simulink library "csc_gnd_sta_lib"  (R2014b)
settings: Solver=ode45  StartTime=0.0  StopTime=10.0  RelTol=1e-3
undefined symbols (not defined in the file): scenario_data_dir
libraries: util_info_lib x1
settings Model: Creator=mstewart  LastModifiedBy=mstewart

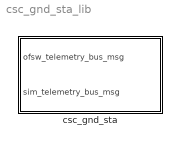
== system csc_gnd_sta_lib ==
  csc_gnd_sta : Subsystem  mask{dir_name=scenario_data_dir}
      mask prompts: dir_name "File Destination Directory (include '')"
      mask init:
      | csc_gnd_sta_callback(gcb, dir_name);
      mask Display:
      | color('blue');
      | text(0.02,0.05,'MoonEx', ...
      |  	'HorizontalAlignment','Left', ...
      | 	'VerticalAlignment','Bottom');

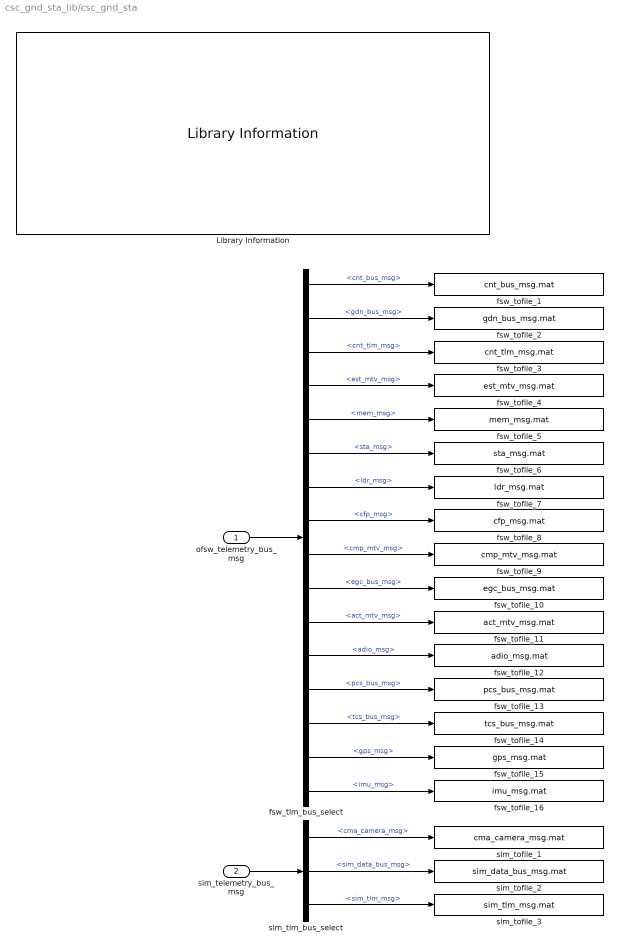
== system csc_gnd_sta_lib/csc_gnd_sta ==
  ofsw_telemetry_bus_msg : Inport
  sim_telemetry_bus_msg : Inport  Port=2
  Library Information : util_info_lib/Library Information  owner='NONE'
  fsw_tlm_bus_select : BusSelector  OutputSignals=cnt_bus_msg,gdn_bus_msg,cnt_tlm_msg,est_mtv_msg,mem_msg,sta_msg,ldr_msg,cfp_msg,cmp_mtv_msg,egc_bus_msg,act_mtv_msg,adio_msg,pcs_bus_msg,tcs_bus_msg,gps_msg,imu_msg
  fsw_tofile_1 : ToFile  Filename=cnt_bus_msg.mat  MatrixName=data  SaveFormat=Timeseries
  fsw_tofile_10 : ToFile  Filename=egc_bus_msg.mat  MatrixName=data  SaveFormat=Timeseries
  fsw_tofile_11 : ToFile  Filename=act_mtv_msg.mat  MatrixName=data  SaveFormat=Timeseries
  fsw_tofile_12 : ToFile  Filename=adio_msg.mat  MatrixName=data  SaveFormat=Timeseries
  fsw_tofile_13 : ToFile  Filename=pcs_bus_msg.mat  MatrixName=data  SaveFormat=Timeseries
  fsw_tofile_14 : ToFile  Filename=tcs_bus_msg.mat  MatrixName=data  SaveFormat=Timeseries
  fsw_tofile_15 : ToFile  Filename=gps_msg.mat  MatrixName=data  SaveFormat=Timeseries
  fsw_tofile_16 : ToFile  Filename=imu_msg.mat  MatrixName=data  SaveFormat=Timeseries
  fsw_tofile_2 : ToFile  Filename=gdn_bus_msg.mat  MatrixName=data  SaveFormat=Timeseries
  fsw_tofile_3 : ToFile  Filename=cnt_tlm_msg.mat  MatrixName=data  SaveFormat=Timeseries
  fsw_tofile_4 : ToFile  Filename=est_mtv_msg.mat  MatrixName=data  SaveFormat=Timeseries
  fsw_tofile_5 : ToFile  Filename=mem_msg.mat  MatrixName=data  SaveFormat=Timeseries
  fsw_tofile_6 : ToFile  Filename=sta_msg.mat  MatrixName=data  SaveFormat=Timeseries
  fsw_tofile_7 : ToFile  Filename=ldr_msg.mat  MatrixName=data  SaveFormat=Timeseries
  fsw_tofile_8 : ToFile  Filename=cfp_msg.mat  MatrixName=data  SaveFormat=Timeseries
  fsw_tofile_9 : ToFile  Filename=cmp_mtv_msg.mat  MatrixName=data  SaveFormat=Timeseries
  sim_tlm_bus_select : BusSelector  OutputSignals=cma_camera_msg,sim_data_bus_msg,sim_tlm_msg
  sim_tofile_1 : ToFile  Filename=cma_camera_msg.mat  MatrixName=data  SaveFormat=Timeseries
  sim_tofile_2 : ToFile  Filename=sim_data_bus_msg.mat  MatrixName=data  SaveFormat=Timeseries
  sim_tofile_3 : ToFile  Filename=sim_tlm_msg.mat  MatrixName=data  SaveFormat=Timeseries
  wires:
  sim_tlm_bus_select/3 -> sim_tofile_3/1  "<sim_tlm_msg>"
  sim_tlm_bus_select/2 -> sim_tofile_2/1  "<sim_data_bus_msg>"
  fsw_tlm_bus_select/16 -> fsw_tofile_16/1  "<imu_msg>"
  fsw_tlm_bus_select/15 -> fsw_tofile_15/1  "<gps_msg>"
  fsw_tlm_bus_select/14 -> fsw_tofile_14/1  "<tcs_bus_msg>"
  fsw_tlm_bus_select/13 -> fsw_tofile_13/1  "<pcs_bus_msg>"
  fsw_tlm_bus_select/12 -> fsw_tofile_12/1  "<adio_msg>"
  fsw_tlm_bus_select/11 -> fsw_tofile_11/1  "<act_mtv_msg>"
  fsw_tlm_bus_select/10 -> fsw_tofile_10/1  "<egc_bus_msg>"
  fsw_tlm_bus_select/9 -> fsw_tofile_9/1  "<cmp_mtv_msg>"
  fsw_tlm_bus_select/8 -> fsw_tofile_8/1  "<cfp_msg>"
  fsw_tlm_bus_select/7 -> fsw_tofile_7/1  "<ldr_msg>"
  fsw_tlm_bus_select/6 -> fsw_tofile_6/1  "<sta_msg>"
  fsw_tlm_bus_select/5 -> fsw_tofile_5/1  "<mem_msg>"
  fsw_tlm_bus_select/4 -> fsw_tofile_4/1  "<est_mtv_msg>"
  fsw_tlm_bus_select/3 -> fsw_tofile_3/1  "<cnt_tlm_msg>"
  fsw_tlm_bus_select/2 -> fsw_tofile_2/1  "<gdn_bus_msg>"
  ofsw_telemetry_bus_msg/1 -> fsw_tlm_bus_select/1
  sim_telemetry_bus_msg/1 -> sim_tlm_bus_select/1
  fsw_tlm_bus_select/1 -> fsw_tofile_1/1  "<cnt_bus_msg>"
  sim_tlm_bus_select/1 -> sim_tofile_1/1  "<cma_camera_msg>"
